simulink model "SSRDDC"  (R2023b)
settings: Solver=VariableStepAuto  StartTime=0.0  StopTime=10E-6  RelTol=1e-3
PreLoadFcn:
  | Fbits=48; %frequency resolution
  | Abits=16; %Sin/COS table depth is 2^Abits
  | Dbits=18; %Sin/COS table width is 1..-Dbits
  | 
  | 
  | clk = 500e+6; % Hz
  | sample_rate = 1/1500e+6; % 1.5GHz
  | SSR = ceil((1/sample_rate)*(1/clk));
  | Tclk = 1/clk;
  | Ts = sample_rate;
  | 
  | % FIR filter chain variables
  | fir0=[-6,0,54,0,-254,0,1230,2048,1230,0,-254,0,54,0,-6];
  | 
  | fir1=[-12,0,84,0,-337,0,1008,0,-2693,0,10142,16384,10142,0,-2693,0,1008,0,-337,0,84,0,-12];
  | 
  | fir2=[5,0,-17,0,44,0,-96,0,187,0,-335,0,565,0,-906,0,1401,0,-2112,0,3145,0,-4723,0,7415,0,-13331,0,41526,65536,41526,0,-13331,0,7415,0,-4723,0,3145,0,-2112,0,1401,0,-906,0,565,0,-335,0,187,0,-96,0,44,0,-17,0,5];
StartFcn:
  | start_time = tic;
StopFcn:
  | stop_time = toc(start_time)/60
libraries: hdlBasic x16, hdlSSR x13, simulink x2, dspsrcs4 x1, hdlUtilities x1, vmcUtilities x1
settings Model: Creator=admin  LastModifiedBy=Jakub
settings SolverCC: AlgebraicLoopSolver=TrustRegion
settings DataIOCC: ReturnWorkspaceOutputs=off
settings DebuggingCC: UnconnectedInputMsg=warning  UnconnectedOutputMsg=warning  UnconnectedLineMsg=warning  ArithmeticOperatorsInVariantConditions=warning
settings ModelReferenceCC: EnableRefExpFcnMdlSchedulingChecks=on
settings SFSimCC: SimUseLocalCustomCode=off  CustomCodeUndefinedFunction=UseInterfaceOnly
settings RTWCC: RTWUseLocalCustomCode=off  DLArmComputeVersion=19.05
settings CodeAppCC: StateflowObjectComments=on

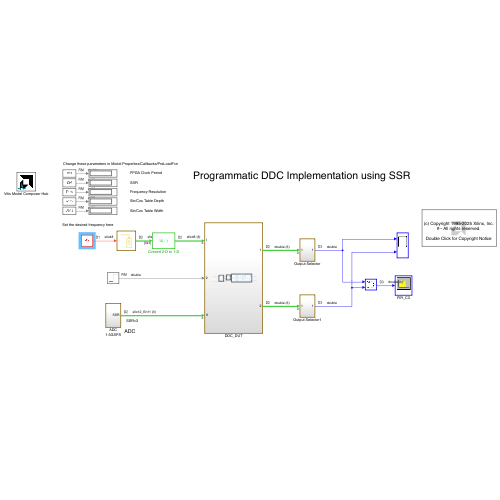
[thumbnail: Simulink's stored preview of the top-level diagram]
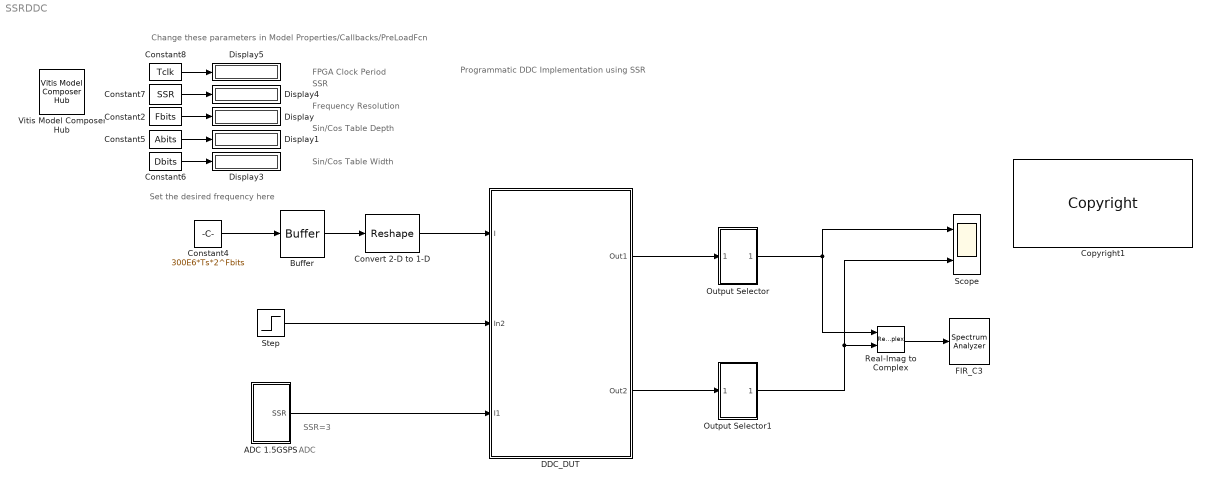
== system SSRDDC ==
  note: Frequency Resolution
  note: Set the desired frequency here
  note: Change these parameters in Model Properties/Callbacks/PreLoadFcn
  note: SSR=3
  note: SSR
  note: FPGA Clock Period
  note: Sin/Cos Table Width
  note: Sin/Cos Table Depth
  note: Programmatic DDC Implementation using SSR
  note: ADC
  ADC 1.5GSPS : Subsystem
  Buffer : Buffer  N=SSR  OutputFrames=off
  Constant2 : Constant  Value=Fbits  OutDataTypeStr=int32  SampleTime=-1
  Constant4 : Constant  Value=300E6*Ts*2^Fbits  OutDataTypeStr=fixdt(1,Fbits,0)  SampleTime=-1
  Constant5 : Constant  Value=Abits  OutDataTypeStr=int32  SampleTime=-1
  Constant6 : Constant  Value=Dbits  OutDataTypeStr=int32  SampleTime=-1
  Constant7 : Constant  Value=SSR  OutDataTypeStr=int32  SampleTime=-1
  Constant8 : Constant  Value=Tclk  OutDataTypeStr=double  SampleTime=-1
  Convert 2-D to 1-D : Reshape
  Copyright1 : hdlUtilities/Copyright  copyrighttext="Copyright (c) 2025  by  Xilinx, Inc. All rights reserved.<br><br>This file contains proprietary, confidential information of Xilinx, Inc., is distributed under license from Xilinx, Inc., and may be used, copied and/or disclosed only pursuant to the terms of a valid license agreement with Xilinx, Inc. Xilinx hereby grants you a license to use this file solely for design, simulation, implementation and creation of design files limited to Xilinx devices or technologies. Use with non-Xilinx devices or technologies is expressly prohibited and immediately terminates your license unless covered by a separate agreement.<br><br>Xilinx is providing this design, code, or information \"as-is\" solely for use in developing programs and solutions for Xilinx devices, with no obligation on the part of Xilinx to provide support. By providing this design, code, or information as one possible implementation of this feature, application or standard, Xilinx is making no representation that this implementation is free from any claims of infringement. You are responsible for obtaining any rights you may require for your implementation. Xilinx expressly disclaims any warranty whatsoever with respect to the adequacy of the implementation, including but not limited to any warranties or representations that this implementation is free from claims of infringement, implied warranties of merchantability or fitness for a particular purpose.<br><br>Xilinx products are not intended for use in life support appliances, devices, or systems. Use in such applications is expressly prohibited.<br><br>Any modifications that are made to the Source Code are done at the user's sole risk and will be unsupported.<br><br>This copyright and support notice must be retained as part of this text at all times. (c) Copyright 1995-2025 Xilinx, Inc. All rights reserved."  block_type=copyright
  DDC_DUT : Subsystem
  Display{,1,3..5} (5 alike) : Display
  FIR_C3 : SpectrumAnalyzer  Method=Welch  AxesScaling=Manual  AveragingMethod=Exponential  ChannelNames="[\"\"]"  DefaultConfigurationName=spbscopes.SpectrumAnalyzerBlockCfg
  Output Selector : Subsystem
  Output Selector1 : Subsystem
  Real-Imag to Complex : RealImagToComplex
  Scope : Scope  NumInputPorts=2
  Step : Step  Time=10/clk  SampleTime=0
  Vitis Model Composer Hub : vmcUtilities/Vitis Model Composer Hub  Tag=genX  CodeGeneration=off  SubsystemName=DDC_DUT  TargetDirectory=./code  exportDesign=off  analyzeDesign=off  validateDesignOnHw=off  ExportType=System Generator  IpVendor=xilinx.com  IpLibrary=hls  IpVersion=1.0  IpHWLanguage=Verilog  AieCompilerOptions={}  AieSimulatorOptions={}  CreateTestbench=off  TestbenchStackSize=10  RunRtlSim=off  RunCSim=off  RunAieSim=off  AieSimTimeout=50000  RunAieSimProfiling=off  LaunchVitisAnalyzer=off  PlotOutput=off  RunX86Sim=off  X86SimTimeout=10  GenHwImage=off  GenLibadfXo=on  GenHwValidationCode=off  PlatformType=Not Specified  HwSystemType=Baremetal  HwValidationTarget=hw  ProjDevice=Zynq UltraScale+ ZCU111 Evaluation Platform (xczu28dr-ffvg1517-2-e)  ProjDevicePart=xczu28dr-ffvg1517-2-e  AIEType=None  SamplePeriod=-1  ClockFrequency=200  DataPathParallelism=1  xilinxfamily=zynquplusRFSOC  part=xczu28dr  speed=-2-e  package=ffvg1517  directory=./netlist\ip\DDC_DUT\src  testbench=off  incr_netlist=off  synthesis_tool=Vivado  clock_wrapper=Clock Enables  dbl_ovrd=According to Block Masks  dcm_input_clock_period=10  sysclk_period=(1e+9)/clk  simulink_period=1/clk  eval_field=0  IPInfoJsonString="{\"HDLSubsystem\":{\"SubsystemName\":\"DDC_DUT\",\"IPName\":\"DDC_DUT\",\"IPLibrary\":\"VMC\",\"IPVendor\":\"User Company\",\"IPVersion\":\"1.0\"}}"  LogFileName=''  NThreads=4
  wires:
  Output Selector1/1(Out1) -> Scope/2, Real-Imag to Complex/2
  Constant4/1 -> Buffer/1
  Output Selector/1(Out1) -> Real-Imag to Complex/1, Scope/1
  Buffer/1 -> Convert 2-D to 1-D/1
  Constant2/1 -> Display/1
  Constant6/1 -> Display3/1
  Constant7/1 -> Display4/1
  Constant8/1 -> Display5/1
  Real-Imag to Complex/1 -> FIR_C3/1
  Constant5/1 -> Display1/1
  Convert 2-D to 1-D/1 -> DDC_DUT/1(I)
  Step/1 -> DDC_DUT/2(In2)
  ADC 1.5GSPS/1(SSR) -> DDC_DUT/3(I1)
  DDC_DUT/1(Out1) -> Output Selector/1(In1)
  DDC_DUT/2(Out2) -> Output Selector1/1(In1)

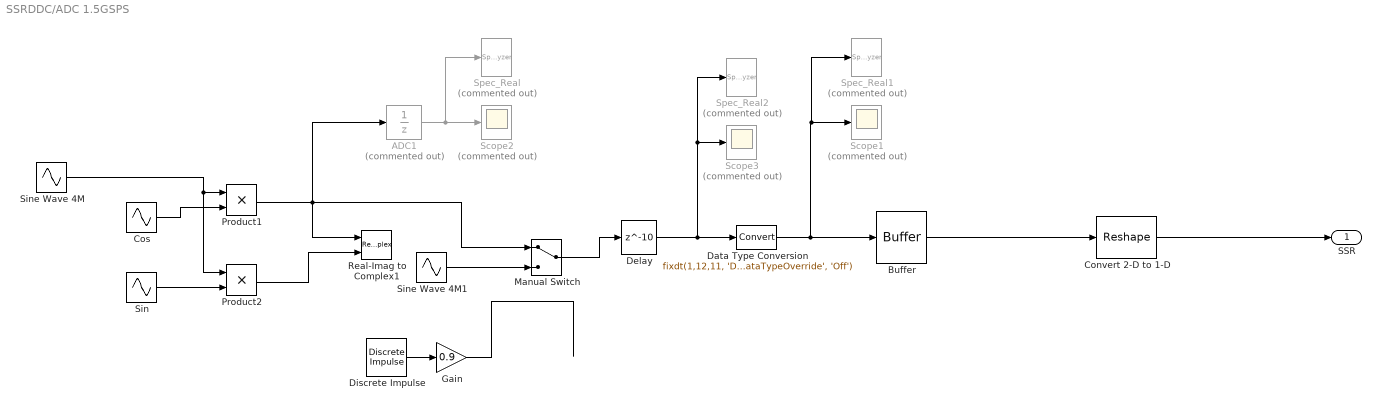
== system SSRDDC/ADC 1.5GSPS ==
  ADC1 : UnitDelay  Commented=on  SampleTime=sample_rate  HasFrameUpgradeWarning=on
  Buffer : Buffer  N=3  OutputFrames=off
  Convert 2-D to 1-D : Reshape
  Cos : Sin  Frequency=300e6*2*pi  Phase=1.5*pi/2  SampleTime=sample_rate
  Data Type Conversion : DataTypeConversion  OutDataTypeStr=fixdt(1,12,11, 'DataTypeOverride', 'Off')  SaturateOnIntegerOverflow=off  RndMeth=Floor  LockScale=on
  Delay : Delay  DelayLength=10  InitialCondition=0
  Discrete Impulse : dspsrcs4/Discrete  Impulse  Delay=1  SampleTime=1/1500e6  FrameSample=1  OutputFrames=off  dataType=double  isSigned=on  wordLen=16  udDataType=sfix(16)  fracBitsMode=Best precision  numFracBits=15  OutDataTypeStr=double  LastOutDataTypeStr=double
  Gain : Gain  Gain=0.9
  Manual Switch : ManualSwitch
  Product1 : Product
  Product2 : Product
  Real-Imag to Complex1 : RealImagToComplex
  Scope1 : Scope  Commented=on
  Scope2 : Scope  Commented=on
  Scope3 : Scope  Commented=on
  Sin : Sin  Frequency=300e6*2*pi  SampleTime=sample_rate
  Sine Wave 4M : Sin  Amplitude=.9  Frequency=4e6*2*pi  SampleTime=sample_rate
  Sine Wave 4M1 : Sin  Amplitude=.9  Frequency=4e6*2*pi  SampleTime=sample_rate
  Spec_Real : SpectrumAnalyzer  Commented=on  WindowPosition=[635.4 8.2 638.4 420]  Method=Welch  SampleRate=1500000000  AxesScaling=Manual  Span=5e-09  StartFrequency=-2.5e-09  StopFrequency=2.5e-09  AveragingMethod=Exponential  YLimits=[-189.2899,40.9275]  ChannelNames="[\"\"]"  DefaultConfigurationName=spbscopes.SpectrumAnalyzerBlockCfg
  Spec_Real1 : SpectrumAnalyzer  Commented=on  WindowPosition=[9 9 1264 630.4]  Method=Welch  SampleRate=1500000000  AxesScaling=Manual  Span=5e-09  StartFrequency=-2.5e-09  StopFrequency=2.5e-09  AveragingMethod=Exponential  YLimits=[-206.5987,41.8342]  ChannelNames="[\"\"]"  DefaultConfigurationName=spbscopes.SpectrumAnalyzerBlockCfg
  Spec_Real2 : SpectrumAnalyzer  Commented=on  WindowPosition=[4.2 13 1264 630.4]  Method=Welch  SampleRate=1500000000  AxesScaling=Manual  Span=5e-09  StartFrequency=-2.5e-09  StopFrequency=2.5e-09  AveragingMethod=Exponential  YLimits=[-206.5987,41.8342]  ChannelNames="[\"\"]"  DefaultConfigurationName=spbscopes.SpectrumAnalyzerBlockCfg
  SSR : Outport  VectorParamsAs1DForOutWhenUnconnected=off
  wires:
  Sine Wave 4M/1 -> Product2/1, Product1/1
  Sin/1 -> Product2/2
  Cos/1 -> Product1/2
  Product1/1 -> Manual Switch/1, Real-Imag to Complex1/1, ADC1/1
  Product2/1 -> Real-Imag to Complex1/2
  ADC1/1 -> Spec_Real/1, Scope2/1
  Buffer/1 -> Convert 2-D to 1-D/1
  Discrete Impulse/1 -> Gain/1
  Sine Wave 4M1/1 -> Manual Switch/2
  Convert 2-D to 1-D/1 -> SSR/1
  Manual Switch/1 -> Delay/1
  Gain/1 -> ?
  Delay/1 -> Data Type Conversion/1, Scope3/1, Spec_Real2/1
  Data Type Conversion/1 -> Buffer/1, Spec_Real1/1, Scope1/1

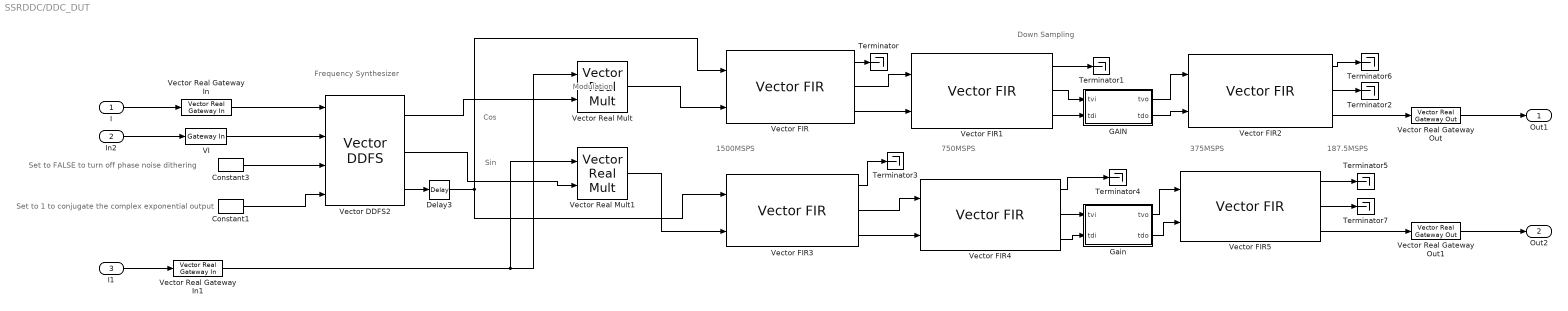
== system SSRDDC/DDC_DUT ==
  note: Down Sampling
  note: Modulation
  note: 187.5MSPS
  note: Set to 1 to conjugate the complex exponential output
  note: Frequency Synthesizer
  note: Cos
  note: Set to FALSE to turn off phase noise dithering
  note: 750MSPS
  note: Sin
  note: 1500MSPS
  note: 375MSPS
  I : Inport
  In2 : Inport  Port=2
  I1 : Inport  Port=3
  Constant1 : hdlBasic/Constant  const=0  gui_display_data_type=Fixed-point  arith_type=Unsigned  n_bits=1  bin_pt=0  preci_type=Single  exp_width=8  frac_width=24  explicit_period=on  period=Tclk  XmcBlockStatus=1  maskContainerNames=tabcontainer1  block_type=constant  block_config=sysgen:Constant_config
  Constant3 : hdlBasic/Constant  const=1  gui_display_data_type=Boolean  arith_type=Boolean  n_bits=1  bin_pt=0  preci_type=Single  exp_width=8  frac_width=24  explicit_period=on  period=Tclk  XmcBlockStatus=1  maskContainerNames=tabcontainer1  block_type=constant  block_config=sysgen:Constant_config
  Delay3 : hdlBasic/Delay  rst=off  en=off  latency=3  reg_retiming=off  XmcBlockStatus=1  maskContainerNames=group1  block_type=delay  block_config=sysgen:Delay_config
  GAIN : Subsystem
      mask Display:
      | fprintf('','COMMENT: begin icon graphics');
      | patch([0 0 3 3 ],[174 92 92 174 ],[6.025000e-01 6.400000e-01 7.075000e-01 ]);
      | patch([0 0 3 3 ],[84 2 2 84 ],[4.350000e-01 4.600000e-01 5.050000e-01 ]);
      | patch([152 152 155 155 ],[169 7 7 169 ],[2.675000e-01 2.800000e-01 3.025000e-01 ]);
      | patch([3 151 151 3 3 ],[0 0 176 176 0 ], [7.700000e-01 8.200000e-01 9.100000e-01 ]);
      | plot([3 151 151 3 3 ],[0 0 176 176 0 ]);
      | 
      | 
      | patch([28.05 59.84 81.84 103.84 125.84 81.84 50.05 28.05 ],[112.42 112.42 134.42 112.42 134.42 134.42 134.42 112.42 ],[1 1 1 ]);
      | patch([50.05 81.84 59.84 28.05 50.05 ],[90.42 90.42 112.42 112.42 90.42 ],[0.931 0.946 0.973 ]);
      | patch([28.05 59.84 81.84 50.05 28.05 ],[68.42 68.42 90.42 90.42 68.42 ],[1 1 1 ]);
      | patch([50.05 125.84 103.84 81.84 59.84 28.05 50.05 ],[46.42 46.42 68.42 46.42 68.42 68.42 46.42 ],[0.931 0.946 0.973 ]);
      | fprintf('','COMMENT: end icon graphics');
      | fprintf('','COMMENT: begin icon text');
      | color('black');port_label('input',1,'\fontsize{11pt}\bf tvi ','texmode','on');
      | color('black');port_label('input',2,'\fontsize{11pt}\bf tdi ','texmode','on');
      | color('black');port_label('output',1,'\fontsize{11pt}\bf tvo ','texmode','on');
      | color('black');port_label('output',2,'\fontsize{11pt}\bf tdo ','texmode','on');
      | fprintf('','COMMENT: end icon text');
  Gain : Subsystem
      mask Display:
      | fprintf('','COMMENT: begin icon graphics');
      | patch([0 0 3 3 ],[174 92 92 174 ],[6.025000e-01 6.400000e-01 7.075000e-01 ]);
      | patch([0 0 3 3 ],[84 2 2 84 ],[4.350000e-01 4.600000e-01 5.050000e-01 ]);
      | patch([152 152 155 155 ],[169 7 7 169 ],[2.675000e-01 2.800000e-01 3.025000e-01 ]);
      | patch([3 151 151 3 3 ],[0 0 176 176 0 ],[7.700000e-01 8.200000e-01 9.100000e-01 ]);
      | plot([3 151 151 3 3 ],[0 0 176 176 0 ]);
      | 
      | 
      | patch([28.05 59.84 81.84 103.84 125.84 81.84 50.05 28.05 ],[112.42 112.42 134.42 112.42 134.42 134.42 134.42 112.42 ],[1 1 1 ]);
      | patch([50.05 81.84 59.84 28.05 50.05 ],[90.42 90.42 112.42 112.42 90.42 ],[0.931 0.946 0.973 ]);
      | patch([28.05 59.84 81.84 50.05 28.05 ],[68.42 68.42 90.42 90.42 68.42 ],[1 1 1 ]);
      | patch([50.05 125.84 103.84 81.84 59.84 28.05 50.05 ],[46.42 46.42 68.42 46.42 68.42 68.42 46.42 ],[0.931 0.946 0.973 ]);
      | fprintf('','COMMENT: end icon graphics');
      | fprintf('','COMMENT: begin icon text');
      | color('black');port_label('input',1,'\fontsize{11pt}\bf tvi ','texmode','on');
      | color('black');port_label('input',2,'\fontsize{11pt}\bf tdi ','texmode','on');
      | color('black');port_label('output',1,'\fontsize{11pt}\bf tvo ','texmode','on');
      | color('black');port_label('output',2,'\fontsize{11pt}\bf tdo ','texmode','on');
      | fprintf('','COMMENT: end icon text');
  Terminator{,1..7} (8 alike) : Terminator
  VI : hdlBasic/Gateway In  gui_display_data_type=Boolean  arith_type=Boolean  n_bits=48  bin_pt=0  preci_type=Single  exp_width=8  frac_width=24  rows=1  columns=1  quantization="Round  (unbiased: +/- Inf)"  overflow=Saturate  period=Tclk  UseAsADC=off  ADCChannel='1'  interface=None  automatic_assignment=on  address_offset=hex2dec('00')  intf_name=''  intf_description=''  default_value=0  timing_constraint=None  locs_specified=off  LOCs={}  io_standard={}  inherit_from_input=off  hdl_port=on  XmcBlockStatus=1  maskContainerNames=group4  block_type=gatewayin  block_config=sysgen:gateway_in_config  block_width_w=590  block_height_w=620  block_width=640  block_height=850
  Vector DDFS2 : hdlSSR/Vector DDFS  sg_ssr=SSR  Fbits=Fbits  Abits=Abits  Dbits=Dbits  block_type=ddfs_ssr  XmcBlockStatus=1  sg_ssr_prev=3  maskContainerNames=group1
  Vector FIR : hdlSSR/Vector FIR  coefficientvector=fir0  coefficient_sets=1  coefficient_reload=off  filter_type=Decimation  rate_change_type=Integer  interpolation_rate=1  decimation_rate=2  zero_pack_factor=1  sg_ssr=SSR  coefficient_sign=Signed  quantization=Integer_Coefficients  coefficient_width=13  bestprecision=off  coefficient_fractional_bits=0  coefficient_structure=Inferred  output_rounding_mode=Truncate_LSBs  output_width=24  filter_architecture=Systolic_Multiply_Accumulate  optimization_goal=Area  optimization_list='None'  data_buffer_type=Automatic  coefficient_buffer_type=Automatic  input_buffer_type=Automatic  output_buffer_type=Automatic  preference_for_other_storage=Automatic  multi_column_support=Automatic  columnconfig='1'  inter_column_pipe_length=4  m_data_has_tready=off  has_aclken=off  has_aresetn=off  reset_data_vector=on  simulation_type=xsim  simulation_model=sysgen:xfirv7_2_cmodel  data_path_portlist={ 's_axis_data_tdata', 'm_axis_data_tdata' }  passband_min=0.0  passband_max=0.5  stopband_min=0.5  stopband_max=1.0  filter_selection=1  gui_behaviour=1  data_sign=Signed  data_width=16  data_fractional_bits=0  data_tuser_width='11'  wrapper_available=true  ip_wrap_arbitrary_binary_point=true  ip_name=FIR Compiler  ip_version=7.2  dsptool_ready=true  ipcore_usecache=true  ipcore_useipmodelcache=true  port_translation_map={ 'aclken' => 'en', 'aresetn' => 'rst' }  run_core_at_system_period=true  ipcore_xco_need_fpga_part=true  ipcore_fpga_part=[]  block_type=fir_compiler_v7_2_ssr  decimation_prev=2  interpolation_prev=1  coeffsets_prev=1  filter_prev=Decimation  channel_sequence=Basic  number_channels=1  pattern_list='P4-0,P4-1,P4-2,P4-3,P4-4'  number_paths=1  data_has_tlast=Not_Required  s_data_has_fifo=off  s_data_has_tuser=Not_Required  m_data_has_tuser=Not_Required  s_config_sync_mode=On_Vector  s_config_method=Single  num_reload_slots=1  XmcBlockStatus=1  sg_ssr_prev=3  maskContainerNames=group10  block_width=657
      settings: block_version=1.0
  Vector FIR1 : hdlSSR/Vector FIR  coefficientvector=fir1  coefficient_sets=1  coefficient_reload=off  filter_type=Decimation  rate_change_type=Integer  interpolation_rate=1  decimation_rate=2  zero_pack_factor=1  sg_ssr=SSR  coefficient_sign=Signed  quantization=Integer_Coefficients  coefficient_width=16  bestprecision=off  coefficient_fractional_bits=0  coefficient_structure=Inferred  output_rounding_mode=Truncate_LSBs  output_width=30  filter_architecture=Systolic_Multiply_Accumulate  optimization_goal=Area  optimization_list='None'  data_buffer_type=Automatic  coefficient_buffer_type=Automatic  input_buffer_type=Automatic  output_buffer_type=Automatic  preference_for_other_storage=Automatic  multi_column_support=Automatic  columnconfig='1'  inter_column_pipe_length=4  m_data_has_tready=off  has_aclken=off  has_aresetn=off  reset_data_vector=on  simulation_type=xsim  simulation_model=sysgen:xfirv7_2_cmodel  data_path_portlist={ 's_axis_data_tdata', 'm_axis_data_tdata' }  passband_min=0.0  passband_max=0.5  stopband_min=0.5  stopband_max=1.0  filter_selection=1  gui_behaviour=1  data_sign=Signed  data_width=16  data_fractional_bits=0  data_tuser_width='11'  wrapper_available=true  ip_wrap_arbitrary_binary_point=true  ip_name=FIR Compiler  ip_version=7.2  dsptool_ready=true  ipcore_usecache=true  ipcore_useipmodelcache=true  port_translation_map={ 'aclken' => 'en', 'aresetn' => 'rst' }  run_core_at_system_period=true  ipcore_xco_need_fpga_part=true  ipcore_fpga_part=[]  block_type=fir_compiler_v7_2_ssr  decimation_prev=2  interpolation_prev=1  coeffsets_prev=1  filter_prev=Decimation  channel_sequence=Basic  number_channels=1  pattern_list='P4-0,P4-1,P4-2,P4-3,P4-4'  number_paths=1  data_has_tlast=Not_Required  s_data_has_fifo=off  s_data_has_tuser=Not_Required  m_data_has_tuser=Not_Required  s_config_sync_mode=On_Vector  s_config_method=Single  num_reload_slots=1  XmcBlockStatus=1  sg_ssr_prev=3  maskContainerNames=group10  block_width=657
      settings: block_version=1.0
  Vector FIR2 : hdlSSR/Vector FIR  coefficientvector=fir2  coefficient_sets=1  coefficient_reload=off  filter_type=Decimation  rate_change_type=Integer  interpolation_rate=1  decimation_rate=2  zero_pack_factor=1  sg_ssr=SSR  coefficient_sign=Signed  quantization=Integer_Coefficients  coefficient_width=18  bestprecision=off  coefficient_fractional_bits=0  coefficient_structure=Inferred  output_rounding_mode=Full_Precision  output_width=30  filter_architecture=Systolic_Multiply_Accumulate  optimization_goal=Area  optimization_list='None'  data_buffer_type=Automatic  coefficient_buffer_type=Automatic  input_buffer_type=Automatic  output_buffer_type=Automatic  preference_for_other_storage=Automatic  multi_column_support=Automatic  columnconfig='1'  inter_column_pipe_length=4  m_data_has_tready=off  has_aclken=off  has_aresetn=off  reset_data_vector=on  simulation_type=xsim  simulation_model=sysgen:xfirv7_2_cmodel  data_path_portlist={ 's_axis_data_tdata', 'm_axis_data_tdata' }  passband_min=0.0  passband_max=0.5  stopband_min=0.5  stopband_max=1.0  filter_selection=1  gui_behaviour=1  data_sign=Signed  data_width=16  data_fractional_bits=0  data_tuser_width='11'  wrapper_available=true  ip_wrap_arbitrary_binary_point=true  ip_name=FIR Compiler  ip_version=7.2  dsptool_ready=true  ipcore_usecache=true  ipcore_useipmodelcache=true  port_translation_map={ 'aclken' => 'en', 'aresetn' => 'rst' }  run_core_at_system_period=true  ipcore_xco_need_fpga_part=true  ipcore_fpga_part=[]  block_type=fir_compiler_v7_2_ssr  decimation_prev=2  interpolation_prev=1  coeffsets_prev=1  filter_prev=Decimation  channel_sequence=Basic  number_channels=1  pattern_list='P4-0,P4-1,P4-2,P4-3,P4-4'  number_paths=1  data_has_tlast=Not_Required  s_data_has_fifo=off  s_data_has_tuser=Not_Required  m_data_has_tuser=Not_Required  s_config_sync_mode=On_Vector  s_config_method=Single  num_reload_slots=1  XmcBlockStatus=1  sg_ssr_prev=3  maskContainerNames=group10  block_width=657
      settings: block_version=1.0
  Vector FIR3 : hdlSSR/Vector FIR  coefficientvector=fir0  coefficient_sets=1  coefficient_reload=off  filter_type=Decimation  rate_change_type=Integer  interpolation_rate=1  decimation_rate=2  zero_pack_factor=1  sg_ssr=SSR  coefficient_sign=Signed  quantization=Integer_Coefficients  coefficient_width=13  bestprecision=off  coefficient_fractional_bits=0  coefficient_structure=Inferred  output_rounding_mode=Truncate_LSBs  output_width=24  filter_architecture=Systolic_Multiply_Accumulate  optimization_goal=Area  optimization_list='None'  data_buffer_type=Automatic  coefficient_buffer_type=Automatic  input_buffer_type=Automatic  output_buffer_type=Automatic  preference_for_other_storage=Automatic  multi_column_support=Automatic  columnconfig='1'  inter_column_pipe_length=4  m_data_has_tready=off  has_aclken=off  has_aresetn=off  reset_data_vector=on  simulation_type=xsim  simulation_model=sysgen:xfirv7_2_cmodel  data_path_portlist={ 's_axis_data_tdata', 'm_axis_data_tdata' }  passband_min=0.0  passband_max=0.5  stopband_min=0.5  stopband_max=1.0  filter_selection=1  gui_behaviour=1  data_sign=Signed  data_width=16  data_fractional_bits=0  data_tuser_width='11'  wrapper_available=true  ip_wrap_arbitrary_binary_point=true  ip_name=FIR Compiler  ip_version=7.2  dsptool_ready=true  ipcore_usecache=true  ipcore_useipmodelcache=true  port_translation_map={ 'aclken' => 'en', 'aresetn' => 'rst' }  run_core_at_system_period=true  ipcore_xco_need_fpga_part=true  ipcore_fpga_part=[]  block_type=fir_compiler_v7_2_ssr  decimation_prev=2  interpolation_prev=1  coeffsets_prev=1  filter_prev=Decimation  channel_sequence=Basic  number_channels=1  pattern_list='P4-0,P4-1,P4-2,P4-3,P4-4'  number_paths=1  data_has_tlast=Not_Required  s_data_has_fifo=off  s_data_has_tuser=Not_Required  m_data_has_tuser=Not_Required  s_config_sync_mode=On_Vector  s_config_method=Single  num_reload_slots=1  XmcBlockStatus=1  sg_ssr_prev=3  maskContainerNames=group10  block_width=657
      settings: block_version=1.0
  Vector FIR4 : hdlSSR/Vector FIR  coefficientvector=fir1  coefficient_sets=1  coefficient_reload=off  filter_type=Decimation  rate_change_type=Integer  interpolation_rate=1  decimation_rate=2  zero_pack_factor=1  sg_ssr=SSR  coefficient_sign=Signed  quantization=Integer_Coefficients  coefficient_width=16  bestprecision=off  coefficient_fractional_bits=0  coefficient_structure=Inferred  output_rounding_mode=Truncate_LSBs  output_width=30  filter_architecture=Systolic_Multiply_Accumulate  optimization_goal=Area  optimization_list='None'  data_buffer_type=Automatic  coefficient_buffer_type=Automatic  input_buffer_type=Automatic  output_buffer_type=Automatic  preference_for_other_storage=Automatic  multi_column_support=Automatic  columnconfig='1'  inter_column_pipe_length=4  m_data_has_tready=off  has_aclken=off  has_aresetn=off  reset_data_vector=on  simulation_type=xsim  simulation_model=sysgen:xfirv7_2_cmodel  data_path_portlist={ 's_axis_data_tdata', 'm_axis_data_tdata' }  passband_min=0.0  passband_max=0.5  stopband_min=0.5  stopband_max=1.0  filter_selection=1  gui_behaviour=1  data_sign=Signed  data_width=16  data_fractional_bits=0  data_tuser_width='11'  wrapper_available=true  ip_wrap_arbitrary_binary_point=true  ip_name=FIR Compiler  ip_version=7.2  dsptool_ready=true  ipcore_usecache=true  ipcore_useipmodelcache=true  port_translation_map={ 'aclken' => 'en', 'aresetn' => 'rst' }  run_core_at_system_period=true  ipcore_xco_need_fpga_part=true  ipcore_fpga_part=[]  block_type=fir_compiler_v7_2_ssr  decimation_prev=2  interpolation_prev=1  coeffsets_prev=1  filter_prev=Decimation  channel_sequence=Basic  number_channels=1  pattern_list='P4-0,P4-1,P4-2,P4-3,P4-4'  number_paths=1  data_has_tlast=Not_Required  s_data_has_fifo=off  s_data_has_tuser=Not_Required  m_data_has_tuser=Not_Required  s_config_sync_mode=On_Vector  s_config_method=Single  num_reload_slots=1  XmcBlockStatus=1  sg_ssr_prev=3  maskContainerNames=group10  block_width=657
      settings: block_version=1.0
  Vector FIR5 : hdlSSR/Vector FIR  coefficientvector=fir2  coefficient_sets=1  coefficient_reload=off  filter_type=Decimation  rate_change_type=Integer  interpolation_rate=1  decimation_rate=2  zero_pack_factor=1  sg_ssr=SSR  coefficient_sign=Signed  quantization=Integer_Coefficients  coefficient_width=18  bestprecision=off  coefficient_fractional_bits=0  coefficient_structure=Inferred  output_rounding_mode=Full_Precision  output_width=30  filter_architecture=Systolic_Multiply_Accumulate  optimization_goal=Area  optimization_list='None'  data_buffer_type=Automatic  coefficient_buffer_type=Automatic  input_buffer_type=Automatic  output_buffer_type=Automatic  preference_for_other_storage=Automatic  multi_column_support=Automatic  columnconfig='1'  inter_column_pipe_length=4  m_data_has_tready=off  has_aclken=off  has_aresetn=off  reset_data_vector=on  simulation_type=xsim  simulation_model=sysgen:xfirv7_2_cmodel  data_path_portlist={ 's_axis_data_tdata', 'm_axis_data_tdata' }  passband_min=0.0  passband_max=0.5  stopband_min=0.5  stopband_max=1.0  filter_selection=1  gui_behaviour=1  data_sign=Signed  data_width=16  data_fractional_bits=0  data_tuser_width='11'  wrapper_available=true  ip_wrap_arbitrary_binary_point=true  ip_name=FIR Compiler  ip_version=7.2  dsptool_ready=true  ipcore_usecache=true  ipcore_useipmodelcache=true  port_translation_map={ 'aclken' => 'en', 'aresetn' => 'rst' }  run_core_at_system_period=true  ipcore_xco_need_fpga_part=true  ipcore_fpga_part=[]  block_type=fir_compiler_v7_2_ssr  decimation_prev=2  interpolation_prev=1  coeffsets_prev=1  filter_prev=Decimation  channel_sequence=Basic  number_channels=1  pattern_list='P4-0,P4-1,P4-2,P4-3,P4-4'  number_paths=1  data_has_tlast=Not_Required  s_data_has_fifo=off  s_data_has_tuser=Not_Required  m_data_has_tuser=Not_Required  s_config_sync_mode=On_Vector  s_config_method=Single  num_reload_slots=1  XmcBlockStatus=1  sg_ssr_prev=3  maskContainerNames=group10  block_width=657
      settings: block_version=1.0
  Vector Real Gateway In : hdlSSR/Vector Real Gateway In  gui_display_data_type=Fixed-point  arith_type=Signed (2's comp)  n_bits=Fbits  bin_pt=0  preci_type=Double  exp_width=80  frac_width=240  quantization=Truncate  overflow=Wrap  period=Tclk  sg_ssr=SSR  UseAsADC=off  ADCChannel='1'  interface=None  automatic_assignment=on  address_offset=hex2dec('00')  intf_name=''  intf_description=''  default_value=0  timing_constraint=None  locs_specified=off  LOCs={}  io_standard={}  inherit_from_input=off  hdl_port=on  interface_prev=1  block_type=gatewayin  XmcBlockStatus=1  sg_ssr_prev=3  maskContainerNames=group4  block_width_w=590  block_height_w=670  block_width=640  block_height=850
  Vector Real Gateway In1 : hdlSSR/Vector Real Gateway In  gui_display_data_type=Fixed-point  arith_type=Signed (2's comp)  n_bits=12  bin_pt=11  preci_type=Single  exp_width=8  frac_width=24  quantization=Truncate  overflow=Wrap  period=1/clk  sg_ssr=SSR  UseAsADC=off  ADCChannel='1'  interface=None  automatic_assignment=on  address_offset=hex2dec('00')  intf_name=''  intf_description=''  default_value=0  timing_constraint=None  locs_specified=off  LOCs={}  io_standard={}  inherit_from_input=off  hdl_port=on  interface_prev=1  block_type=gatewayin  XmcBlockStatus=1  sg_ssr_prev=3  maskContainerNames=group4  block_width_w=590  block_height_w=670  block_width=640  block_height=850
  Vector Real Gateway Out : hdlSSR/Vector Real Gateway Out  inherit_from_input=off  hdl_port=on  sg_ssr=SSR  rows=1  columns=1  UseAsDAC=off  DACChannel='1'  interface=None  automatic_assignment=on  address_offset=hex2dec('00')  intf_name=''  intf_description=''  timing_constraint=None  locs_specified=off  LOCs={}  io_standard={}  block_type=realgatewayout_ssr  XmcBlockStatus=1  sg_ssr_prev=3  maskContainerNames=group4  block_width_w=590  block_height_w=620  block_width=620  block_height=750
  Vector Real Gateway Out1 : hdlSSR/Vector Real Gateway Out  inherit_from_input=off  hdl_port=on  sg_ssr=SSR  rows=1  columns=1  UseAsDAC=off  DACChannel='1'  interface=None  automatic_assignment=on  address_offset=hex2dec('00')  intf_name=''  intf_description=''  timing_constraint=None  locs_specified=off  LOCs={}  io_standard={}  block_type=realgatewayout_ssr  XmcBlockStatus=1  sg_ssr_prev=3  maskContainerNames=group4  block_width_w=590  block_height_w=620  block_width=620  block_height=750
  Vector Real Mult : hdlSSR/Vector Real Mult  precision=User Defined  arith_type="Signed  (2's comp)"  n_bits=24  bin_pt=22  quantization=Truncate  overflow=Wrap  en=off  sg_latency=3  sg_ssr=SSR  use_behavioral_HDL=off  opt=Speed  use_embedded=on  optimum_pipeline=off  pipeline=on  use_rpm=on  placement_style=Triangular  block_type=realmult_ssr  XmcBlockStatus=1  sg_ssr_prev=3  maskContainerNames=group1
  Vector Real Mult1 : hdlSSR/Vector Real Mult  precision=User Defined  arith_type="Signed  (2's comp)"  n_bits=24  bin_pt=22  quantization=Truncate  overflow=Wrap  en=off  sg_latency=3  sg_ssr=SSR  use_behavioral_HDL=off  opt=Speed  use_embedded=on  optimum_pipeline=off  pipeline=on  use_rpm=on  placement_style=Triangular  block_type=realmult_ssr  XmcBlockStatus=1  sg_ssr_prev=3  maskContainerNames=group1
  Out1 : Outport
  Out2 : Outport  Port=2
  wires:
  Vector FIR5/1 -> Terminator5/1
  Vector FIR1/1 -> Terminator1/1
  Vector FIR4/1 -> Terminator4/1
  Vector FIR5/2 -> Terminator7/1
  Constant1/1 -> Vector DDFS2/4
  Vector DDFS2/3 -> Delay3/1
  Vector FIR3/2 -> Vector FIR4/1
  GAIN/2(tdo) -> Vector FIR2/2
  Vector Real Gateway Out/1 -> Out1/1
  Vector DDFS2/1 -> Vector Real Mult/2
  GAIN/1(tvo) -> Vector FIR2/1
  Vector Real Mult1/1 -> Vector FIR3/2
  Vector Real Mult/1 -> Vector FIR/2
  Vector Real Gateway In1/1 -> Vector Real Mult/1, Vector Real Mult1/1
  I1/1 -> Vector Real Gateway In1/1
  In2/1 -> VI/1
  Vector Real Gateway Out1/1 -> Out2/1
  Vector DDFS2/2 -> Vector Real Mult1/2
  VI/1 -> Vector DDFS2/2
  Vector FIR/1 -> Terminator/1
  Constant3/1 -> Vector DDFS2/3
  Vector FIR2/1 -> Terminator6/1
  Delay3/1 -> Vector FIR/1, Vector FIR3/1
  I/1 -> Vector Real Gateway In/1
  Vector Real Gateway In/1 -> Vector DDFS2/1
  Gain/1(tvo) -> Vector FIR5/1
  Vector FIR5/3 -> Vector Real Gateway Out1/1
  Vector FIR1/2 -> GAIN/1(tvi)
  Vector FIR1/3 -> GAIN/2(tdi)
  Vector FIR3/3 -> Vector FIR4/2
  Vector FIR3/1 -> Terminator3/1
  Vector FIR2/3 -> Vector Real Gateway Out/1
  Vector FIR4/3 -> Gain/2(tdi)
  Vector FIR2/2 -> Terminator2/1
  Vector FIR/3 -> Vector FIR1/2
  Vector FIR4/2 -> Gain/1(tvi)
  Gain/2(tdo) -> Vector FIR5/2
  Vector FIR/2 -> Vector FIR1/1

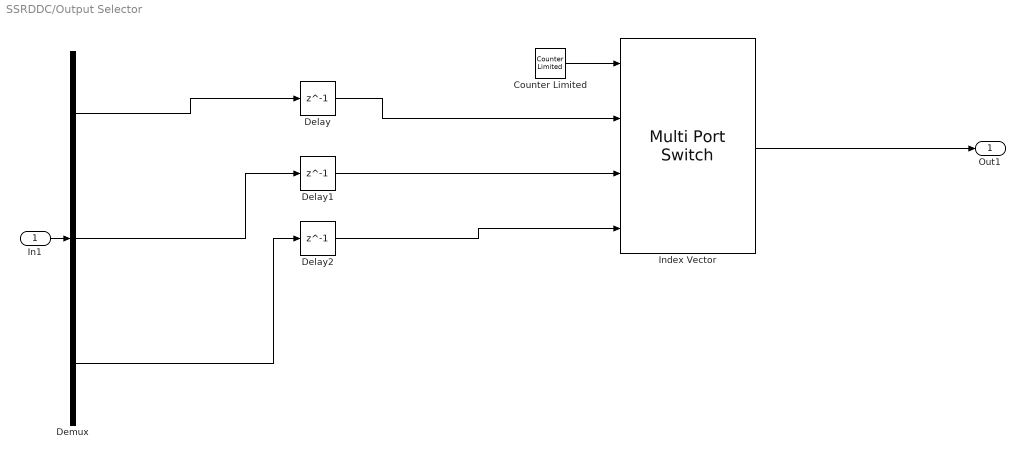
== system SSRDDC/Output Selector ==
  In1 : Inport
  Counter Limited : simulink/Sources/Counter Limited  uplimit=2  tsamp=1/187.5e6
  Delay : Delay  DelayLength=1  InitialCondition=0  SampleTime=1/62.5e6
  Delay1 : Delay  DelayLength=1  InitialCondition=0  SampleTime=1/62.5e6
  Delay2 : Delay  DelayLength=1  InitialCondition=0  SampleTime=1/62.5e6
  Demux : Demux  Outputs=3
  Index Vector : MultiPortSwitch  DataPortOrder=Zero-based contiguous  zeroidx=on  SaturateOnIntegerOverflow=off  InputSameDT=off
  Out1 : Outport  VectorParamsAs1DForOutWhenUnconnected=off
  wires:
  Demux/3 -> Delay2/1
  Index Vector/1 -> Out1/1
  Demux/1 -> Delay/1
  Counter Limited/1 -> Index Vector/1
  Demux/2 -> Delay1/1
  In1/1 -> Demux/1
  Delay1/1 -> Index Vector/3
  Delay2/1 -> Index Vector/4
  Delay/1 -> Index Vector/2

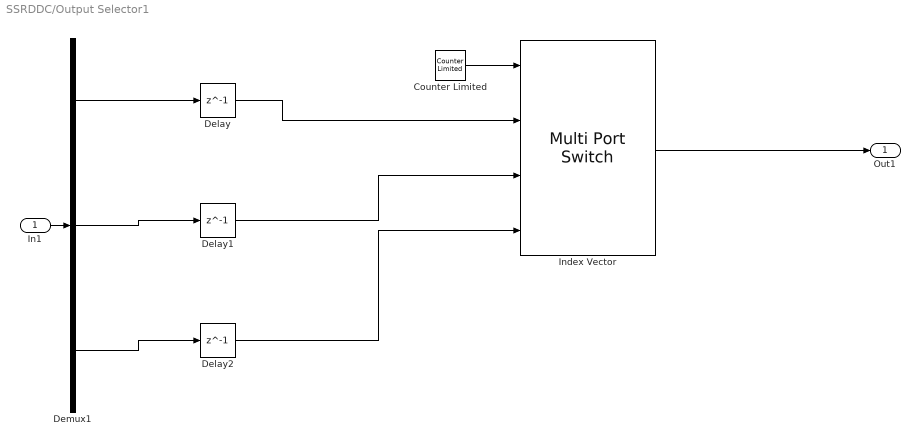
== system SSRDDC/Output Selector1 ==
  In1 : Inport
  Counter Limited : simulink/Sources/Counter Limited  uplimit=2  tsamp=1/187.5e6
  Delay : Delay  DelayLength=1  InitialCondition=0  SampleTime=1/62.5e6
  Delay1 : Delay  DelayLength=1  InitialCondition=0  SampleTime=1/62.5e6
  Delay2 : Delay  DelayLength=1  InitialCondition=0  SampleTime=1/62.5e6
  Demux1 : Demux  Outputs=3
  Index Vector : MultiPortSwitch  DataPortOrder=Zero-based contiguous  zeroidx=on  SaturateOnIntegerOverflow=off  InputSameDT=off
  Out1 : Outport  VectorParamsAs1DForOutWhenUnconnected=off
  wires:
  Demux1/2 -> Delay1/1
  Counter Limited/1 -> Index Vector/1
  In1/1 -> Demux1/1
  Demux1/3 -> Delay2/1
  Delay/1 -> Index Vector/2
  Delay2/1 -> Index Vector/4
  Index Vector/1 -> Out1/1
  Delay1/1 -> Index Vector/3
  Demux1/1 -> Delay/1

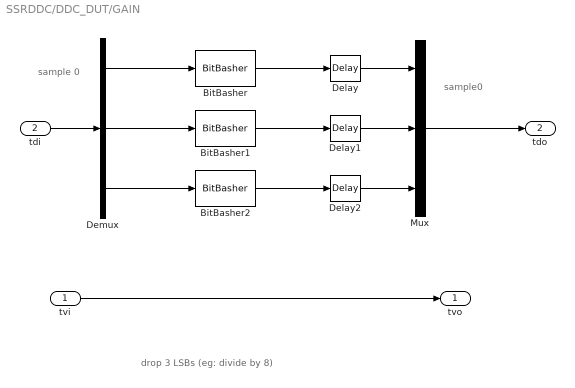
== system SSRDDC/DDC_DUT/GAIN ==
  note: drop 3 LSBs (eg: divide by 8)
  note: sample0
  note: sample 0
  tvi : Inport
  tdi : Inport  Port=2
  BitBasher : hdlBasic/BitBasher  bitexpr=a={c[29:3]}  display_expr=off  sr_1=a  arith_type1="Signed  (2's comp)"  bin_pt1=0  sr_2=2  arith_type2=Unsigned  bin_pt2=0  sr_3=3  arith_type3=Unsigned  bin_pt3=0  sr_4=4  arith_type4=Unsigned  bin_pt4=0  XmcBlockStatus=1  maskContainerNames=group1  block_type=bitbasher  block_config=sysgen:BitBasher_config
  BitBasher1 : hdlBasic/BitBasher  bitexpr=a={c[29:3]}  display_expr=off  sr_1=a  arith_type1="Signed  (2's comp)"  bin_pt1=0  sr_2=2  arith_type2=Unsigned  bin_pt2=0  sr_3=3  arith_type3=Unsigned  bin_pt3=0  sr_4=4  arith_type4=Unsigned  bin_pt4=0  XmcBlockStatus=1  maskContainerNames=group1  block_type=bitbasher  block_config=sysgen:BitBasher_config
  BitBasher2 : hdlBasic/BitBasher  bitexpr=a={c[29:3]}  display_expr=off  sr_1=a  arith_type1="Signed  (2's comp)"  bin_pt1=0  sr_2=2  arith_type2=Unsigned  bin_pt2=0  sr_3=3  arith_type3=Unsigned  bin_pt3=0  sr_4=4  arith_type4=Unsigned  bin_pt4=0  XmcBlockStatus=1  maskContainerNames=group1  block_type=bitbasher  block_config=sysgen:BitBasher_config
  Delay : hdlBasic/Delay  rst=off  en=off  latency=1  reg_retiming=off  XmcBlockStatus=1  maskContainerNames=group1  block_type=delay  block_config=sysgen:Delay_config
  Delay1 : hdlBasic/Delay  rst=off  en=off  latency=1  reg_retiming=off  XmcBlockStatus=1  maskContainerNames=group1  block_type=delay  block_config=sysgen:Delay_config
  Delay2 : hdlBasic/Delay  rst=off  en=off  latency=1  reg_retiming=off  XmcBlockStatus=1  maskContainerNames=group1  block_type=delay  block_config=sysgen:Delay_config
  Demux : Demux  Outputs=3
  Mux : Mux  Inputs=3
  tvo : Outport  VectorParamsAs1DForOutWhenUnconnected=off
  tdo : Outport  Port=2  VectorParamsAs1DForOutWhenUnconnected=off
  wires:
  Mux/1 -> tdo/1
  tdi/1 -> Demux/1
  Demux/1 -> BitBasher/1
  Demux/2 -> BitBasher1/1
  Demux/3 -> BitBasher2/1
  BitBasher2/1 -> Delay2/1
  BitBasher1/1 -> Delay1/1
  tvi/1 -> tvo/1
  BitBasher/1 -> Delay/1
  Delay/1 -> Mux/1
  Delay1/1 -> Mux/2
  Delay2/1 -> Mux/3

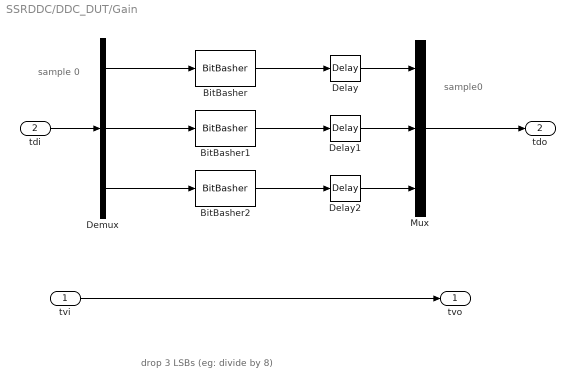
== system SSRDDC/DDC_DUT/Gain ==
  note: drop 3 LSBs (eg: divide by 8)
  note: sample0
  note: sample 0
  tvi : Inport
  tdi : Inport  Port=2
  BitBasher : hdlBasic/BitBasher  bitexpr=a={c[29:3]}  display_expr=off  sr_1=a  arith_type1="Signed  (2's comp)"  bin_pt1=0  sr_2=2  arith_type2=Unsigned  bin_pt2=0  sr_3=3  arith_type3=Unsigned  bin_pt3=0  sr_4=4  arith_type4=Unsigned  bin_pt4=0  XmcBlockStatus=1  maskContainerNames=group1  block_type=bitbasher  block_config=sysgen:BitBasher_config
  BitBasher1 : hdlBasic/BitBasher  bitexpr=a={c[29:3]}  display_expr=off  sr_1=a  arith_type1="Signed  (2's comp)"  bin_pt1=0  sr_2=2  arith_type2=Unsigned  bin_pt2=0  sr_3=3  arith_type3=Unsigned  bin_pt3=0  sr_4=4  arith_type4=Unsigned  bin_pt4=0  XmcBlockStatus=1  maskContainerNames=group1  block_type=bitbasher  block_config=sysgen:BitBasher_config
  BitBasher2 : hdlBasic/BitBasher  bitexpr=a={c[29:3]}  display_expr=off  sr_1=a  arith_type1="Signed  (2's comp)"  bin_pt1=0  sr_2=2  arith_type2=Unsigned  bin_pt2=0  sr_3=3  arith_type3=Unsigned  bin_pt3=0  sr_4=4  arith_type4=Unsigned  bin_pt4=0  XmcBlockStatus=1  maskContainerNames=group1  block_type=bitbasher  block_config=sysgen:BitBasher_config
  Delay : hdlBasic/Delay  rst=off  en=off  latency=1  reg_retiming=off  XmcBlockStatus=1  maskContainerNames=group1  block_type=delay  block_config=sysgen:Delay_config
  Delay1 : hdlBasic/Delay  rst=off  en=off  latency=1  reg_retiming=off  XmcBlockStatus=1  maskContainerNames=group1  block_type=delay  block_config=sysgen:Delay_config
  Delay2 : hdlBasic/Delay  rst=off  en=off  latency=1  reg_retiming=off  XmcBlockStatus=1  maskContainerNames=group1  block_type=delay  block_config=sysgen:Delay_config
  Demux : Demux  Outputs=3
  Mux : Mux  Inputs=3
  tvo : Outport  VectorParamsAs1DForOutWhenUnconnected=off
  tdo : Outport  Port=2  VectorParamsAs1DForOutWhenUnconnected=off
  wires:
  Mux/1 -> tdo/1
  tdi/1 -> Demux/1
  Demux/1 -> BitBasher/1
  Demux/2 -> BitBasher1/1
  Demux/3 -> BitBasher2/1
  BitBasher2/1 -> Delay2/1
  BitBasher1/1 -> Delay1/1
  tvi/1 -> tvo/1
  BitBasher/1 -> Delay/1
  Delay/1 -> Mux/1
  Delay1/1 -> Mux/2
  Delay2/1 -> Mux/3
